simulink model "dspmultichannelhdl"  (Simulink 8.3)
settings: Solver=FixedStepDiscrete  SolverMode=SingleTasking  StartTime=0.0  StopTime=0.5  RelTol=1e-3
InitFcn:
  | Fpass = 0.2; % Passband Frequency
  | Fstop = 0.3; % Stopband Frequency
  | Apass = 1;    % Passband Attenuation (dB)
  | Astop = 60;   % Stopband Attenuation (dB)
  | 
  | f = fdesign.lowpass('Fp,Fst,Ap,Ast',Fpass,Fstop,Apass,Astop);
  | Hlp = design(f, 'equiripple','FilterStructure', 'dffir'); % Lowpass
  | Numerator = Hlp.Numerator;  % coefficients of lowpass filter
libraries: dspsrcs4 x2, dspmisc x1, simulink x1
settings Model: Creator=The MathWorks Inc.
settings DataIOCC: SignalLoggingSaveFormat=Dataset
settings OptimizationCC: ExpressionDepthLimit=2147483647
settings DebuggingCC: ParameterPrecisionLossMsg=none
settings HardwareCC: ProdHWDeviceType=ASIC/FPGA->ASIC/FPGA  TargetBitPerLong=64  TargetBitPerPointer=64  TargetLongLongMode=on  TargetIntDivRoundTo=Zero  TargetEndianess=LittleEndian  TargetWordSize=64  TargetHWDeviceType=Generic->MATLAB Host Computer  ProdEqTarget=off
settings GRTTargetCC: CombineOutputUpdateFcns=on  GRTInterface=off

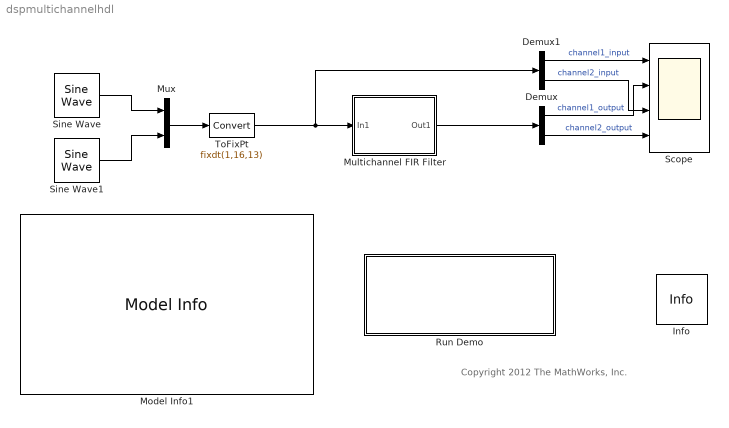
== system dspmultichannelhdl ==
  note: Copyright 2012 The MathWorks, Inc.
  Demux : Demux  Outputs=2
  Demux1 : Demux  Outputs=2
  Info : dspmisc/Info  SystemSampleTime=-1
  Model Info1 : simulink/Model-Wide Utilities/Model Info  InitialBlockCM=None  BlockCM=None  Frame=on  DisplayStringWithTags=|  HorizontalTextAlignment=Left  LeftAlignmentValue=0.02  SourceBlockDiagram=dspmultichannelhdl  TagMaxNumber=20
      | Multichannel FIR Filter
      | 
      | This model shows a FIR filter which 
      | processes multiple input data streams.
      | Specify the 'ChannelSharing' option in
      | HDL Block Properties.
      | 
      | Use the Model Properties initFcn
      | Callback function to set the filter
      | coefficients.
  Multichannel FIR Filter : Subsystem
  Mux : Mux  Inputs=2
  Run Demo : Subsystem
      settings: OpenFcn=hdldialog(bdroot)
      mask Display: disp('Launch HDL Dialog')
  Scope : Scope  NumInputPorts=4
      settings: TimeRange=0.5  YMin=-1~-1~-1~-1  YMax=1~1~1~1
  Sine Wave : dspsrcs4/Sine Wave  Amplitude=1  Frequency=100  Phase=0  SampleMode=Discrete  OutComplex=Real  CompMethod=Trigonometric fcn  TableSize=Speed  SampleTime=1/2000  SamplesPerFrame=1  ResetState=Restart at time zero  dataType=double  wordLen=16  udDataType=sfix(16)  fracBitsMode=Best precision  numFracBits=15  OutDataTypeStr=double  LastOutDataTypeStr=double
  Sine Wave1 : dspsrcs4/Sine Wave  Amplitude=1  Frequency=400  Phase=0  SampleMode=Discrete  OutComplex=Real  CompMethod=Trigonometric fcn  TableSize=Speed  SampleTime=1/2000  SamplesPerFrame=1  ResetState=Restart at time zero  dataType=double  wordLen=16  udDataType=sfix(16)  fracBitsMode=Best precision  numFracBits=15  OutDataTypeStr=double  LastOutDataTypeStr=double
  ToFixPt : DataTypeConversion  OutDataTypeStr=fixdt(1,16,13)
  wires:
  Mux/1 -> ToFixPt/1
  Sine Wave/1 -> Mux/1
  Demux1/1 -> Scope/1  "channel1_input"
  Demux1/2 -> Scope/3  "channel2_input"
  Demux/2 -> Scope/4  "channel2_output"
  ToFixPt/1 -> Demux1/1, Multichannel FIR Filter/1(In1)
  Multichannel FIR Filter/1(Out1) -> Demux/1
  Sine Wave1/1 -> Mux/2
  Demux/1 -> Scope/2  "channel1_output"

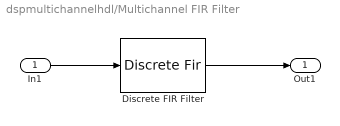
== system dspmultichannelhdl/Multichannel FIR Filter ==
  In1 : Inport
  Discrete FIR Filter : DiscreteFir  FilterStructure=Direct form symmetric  Coefficients=Numerator
  Out1 : Outport
  wires:
  In1/1 -> Discrete FIR Filter/1
  Discrete FIR Filter/1 -> Out1/1

== system dspmultichannelhdl/Run Demo ==
